simulink model "PubIfDecisionTOS_MDL"  (R2020b)
settings: configuration reference "DspaceConfig" (kept outside this file)
PostLoadFcn:
  | if any(exist('dsrtsu_mdlpostloadfcn', 'file') ~= 0), dsrtsu_mdlpostloadfcn('Execute', bdroot); end
InitFcn:
  | , if any(exist('dsmpb_private', 'file') ~= 0), dsmpb_private('dsmpb_mdlclblib', 'Init', bdroot); end,
undefined symbols (not defined in the file or in its folder): C_TOS_ACCEgoRAxletoFbumplength_m, C_TOS_ACCTargetFront_Flag, C_TOS_AEBJAPedObjDxThre_Val, C_TOS_AEBJAPedObjDyThre_Val, C_TOS_AEBJATargetSize_Val, C_TOS_AEBJAVehObjDxThre_Val, C_TOS_AEBJAVehObjDyThre_Val, C_TOS_AEBJuncPedTargetSize_Val, C_TOS_AEBLatObjDxThre_Val, C_TOS_AEBLatPedDyThre_Val, C_TOS_AEBLatTargetSize_Val, C_TOS_AEBLongTargetInEgoFront_Flag, C_TOS_axAbsGround_Parameter, C_TOS_CameraConfirmedFlag, C_TOS_CNsubjWidth, C_TOS_CurrentLaneCoreMinWidth_Val, C_TOS_CutInProb_Val_Zero, C_TOS_CutOutProb_Val_Zero, C_TOS_D2R_Val, C_TOS_DefaultValueObjectToCenterLine_dy, C_TOS_EgoCarWidth_Val, C_TOS_EgoDxRefPoint_m, C_TOS_EgoRAxletoFbumplength_m, C_TOS_HalfWidthVehicle_Con, C_TOS_HWA_CurrentLaneFlag, C_TOS_HWA_LeftLaneFlag, C_TOS_HWA_MovingDir_Vaild, C_TOS_HWA_MovState_Vaild, C_TOS_HWA_RightLaneFlag, C_TOS_LaneLineCourseErrorFront, C_TOS_LaneLineCourseErrorRear, C_TOS_MotorbikeDefaultWidth_m, C_TOS_NumberOfEffectiveTargets, C_TOS_Obj_Age_Val, C_TOS_Objdx_Constraint_Val, C_TOS_ObjectDefaultWidth_m, C_TOS_ObjInCurrentLane_Val, C_TOS_ObjInCurrentLaneValid, C_TOS_ObjInLeftLaneValid, C_TOS_ObjInRightLaneValid, C_TOS_ObjNotInCurrentLane_Val, C_TOS_ObjNotREElementType, C_TOS_ObjPredictDis_dy_ConstantVal_Zeros, C_TOS_ObjToCenterLine_ConstantVal_Zeros, C_TOS_OFMObjIDInvilad_Val, C_TOS_PIL_LatDisCons_Val_zero, C_TOS_PIL_ObjectCutInFlag_b, C_TOS_PIL_ObjectCutOutFlag_b, C_TOS_PIL_ObjLaneProb_al_Val, C_TOS_PP_ObjFusType_FC_Confirm_b, C_TOS_PP_ObjFusType_FC_FR_Confirm_b, C_TOS_PP_ObjFusType_FR_Confirm_b, C_TOS_RE_80BoolDefault_Val, C_TOS_RE_80Single181Default_Val, C_TOS_RE_80Single255Default_Val, C_TOS_RE_80Uint8Default_Val, C_TOS_RE_D2R, C_TOS_RE_D_180_Val, C_TOS_RE_InvalidObjectID_Val, C_TOS_RE_InvalidTargetChainDir_Val ... (+142)
libraries: simulink x1650, TOS_LIB x361, canfdmsglib x14
(part 25 of 69)

== system PubIfDecisionTOS_MDL/TOS_20201112/TOS_2012080320/PP1128/AAT-AdditionalAttributes/PP_SignalProcessing/PP_SignalProcessing/MovingState_SignalProcessing/MovingState_SignalProcessing_V2011120315 ==
  Object_MovingState : Inport
  Compare To Constant : simulink/Logic and Bit Operations/Compare To Constant  relop===  const=OFM_OBJ_MOVINGSTATE_E.MOVING  OutDataTypeStr=boolean
      settings: AttributesFormatString=OFM_OBJ_MOVINGSTATE_E.MOVING = 2
  Compare To Constant1 : simulink/Logic and Bit Operations/Compare To Constant  relop===  const=OFM_OBJ_MOVINGSTATE_E.MOVING_SLOWLY  OutDataTypeStr=boolean
      settings: AttributesFormatString=OFM_OBJ_MOVINGSTATE_E.MOVING_SLOWLY = 5
  Compare To Constant2 : simulink/Logic and Bit Operations/Compare To Constant  relop===  const=OFM_OBJ_MOVINGSTATE_E.STATIONARY  OutDataTypeStr=boolean
      settings: AttributesFormatString=OFM_OBJ_MOVINGSTATE_E.STATIONARY = 3
  Compare To Constant3 : simulink/Logic and Bit Operations/Compare To Constant  relop===  const=OFM_OBJ_MOVINGSTATE_E.STOPPED  OutDataTypeStr=boolean
      settings: AttributesFormatString=OFM_OBJ_MOVINGSTATE_E.STOPPED = 4
  Data Type Conversion : DataTypeConversion  OutDataTypeStr=Enum: OFM_OBJ_MOVINGSTATE_E
  Data Type Conversion1 : DataTypeConversion  OutDataTypeStr=uint8
  Enumerated Constant : simulink/Sources/Enumerated Constant  OutDataTypeStr=Enum: ObjectMovingState_AEB_E  Value=ObjectMovingState_AEB_E.Moving  SampleTime=inf
      settings: AttributesFormatString=ObjectMovingState.Moving =2
  Enumerated Constant1 : simulink/Sources/Enumerated Constant  OutDataTypeStr=Enum: ObjectMovingState_AEB_E  Value=ObjectMovingState_AEB_E.Still  SampleTime=inf
      settings: AttributesFormatString=ObjectMovingState.Still = 1
  Enumerated Constant2 : simulink/Sources/Enumerated Constant  OutDataTypeStr=Enum: ObjectMovingState_AEB_E  Value=ObjectMovingState_AEB_E.Stopped  SampleTime=inf
      settings: AttributesFormatString=ObjectMovingState.Stopped = 3
  Enumerated Constant3 : simulink/Sources/Enumerated Constant  OutDataTypeStr=Enum: ObjectMovingState_AEB_E  Value=ObjectMovingState_AEB_E.UnknownState  SampleTime=inf
      settings: AttributesFormatString=ObjectMovingState.UnknownState = 0
  Logical Operator : Logic  Operator=OR  AllPortsSameDT=off  OutDataTypeStr=boolean
  Switch : Switch  Criteria=u2 ~= 0
  Switch1 : Switch  Criteria=u2 ~= 0
  Switch2 : Switch  Criteria=u2 ~= 0
  PP_MovingStateSignalProcessing : Outport
  wires:
  Switch1/1 -> Switch/3
  Switch2/1 -> Switch1/3
  Enumerated Constant2/1 -> Switch2/1
  Compare To Constant3/1 -> Switch2/2
  Enumerated Constant1/1 -> Switch1/1
  Compare To Constant2/1 -> Switch1/2
  Enumerated Constant/1 -> Switch/1
  Logical Operator/1 -> Switch/2
  Compare To Constant1/1 -> Logical Operator/2
  Compare To Constant/1 -> Logical Operator/1
  Data Type Conversion/1 -> Compare To Constant3/1, Compare To Constant2/1, Compare To Constant1/1, Compare To Constant/1
  Object_MovingState/1 -> Data Type Conversion/1
  Data Type Conversion1/1 -> PP_MovingStateSignalProcessing/1
  Switch/1 -> Data Type Conversion1/1
  Enumerated Constant3/1 -> Switch2/3

== system PubIfDecisionTOS_MDL/TOS_20201112/TOS_2012080320/PP1128/AAT-AdditionalAttributes/PP_SignalProcessing/PP_SignalProcessing/MovingState_SignalProcessing/MovingState_SignalProcessing_V2011130316 ==
  Object_MovingState : Inport
  Compare To Constant : simulink/Logic and Bit Operations/Compare To Constant  relop===  const=OFM_OBJ_MOVINGSTATE_E.MOVING  OutDataTypeStr=boolean
      settings: AttributesFormatString=OFM_OBJ_MOVINGSTATE_E.MOVING = 2
  Compare To Constant1 : simulink/Logic and Bit Operations/Compare To Constant  relop===  const=OFM_OBJ_MOVINGSTATE_E.MOVING_SLOWLY  OutDataTypeStr=boolean
      settings: AttributesFormatString=OFM_OBJ_MOVINGSTATE_E.MOVING_SLOWLY = 5
  Compare To Constant2 : simulink/Logic and Bit Operations/Compare To Constant  relop===  const=OFM_OBJ_MOVINGSTATE_E.STATIONARY  OutDataTypeStr=boolean
      settings: AttributesFormatString=OFM_OBJ_MOVINGSTATE_E.STATIONARY = 3
  Compare To Constant3 : simulink/Logic and Bit Operations/Compare To Constant  relop===  const=OFM_OBJ_MOVINGSTATE_E.STOPPED  OutDataTypeStr=boolean
      settings: AttributesFormatString=OFM_OBJ_MOVINGSTATE_E.STOPPED = 4
  Compare To Constant4 : simulink/Logic and Bit Operations/Compare To Constant  relop===  const=OFM_OBJ_MOVINGSTATE_E.INVALID  OutDataTypeStr=boolean
      settings: AttributesFormatString=OFM_OBJ_MOVINGSTATE_E.INVALID = 0
  Data Type Conversion : DataTypeConversion  OutDataTypeStr=Enum: OFM_OBJ_MOVINGSTATE_E
  Data Type Conversion1 : DataTypeConversion  OutDataTypeStr=uint8
  Enumerated Constant : simulink/Sources/Enumerated Constant  OutDataTypeStr=Enum: ObjectMovingState_E  Value=ObjectMovingState_E.Moving  SampleTime=inf
      settings: AttributesFormatString=ObjectMovingState.Moving =2
  Enumerated Constant1 : simulink/Sources/Enumerated Constant  OutDataTypeStr=Enum: ObjectMovingState_E  Value=ObjectMovingState_E.Still  SampleTime=inf
      settings: AttributesFormatString=ObjectMovingState.Still = 3
  Enumerated Constant2 : simulink/Sources/Enumerated Constant  OutDataTypeStr=Enum: ObjectMovingState_E  Value=ObjectMovingState_E.Stopped  SampleTime=inf
      settings: AttributesFormatString=ObjectMovingState.Stopped = 4
  Enumerated Constant3 : simulink/Sources/Enumerated Constant  OutDataTypeStr=Enum: ObjectMovingState_E  Value=ObjectMovingState_E.UnknownState  SampleTime=inf
      settings: AttributesFormatString=ObjectMovingState.UnknownState = 1
  Enumerated Constant4 : simulink/Sources/Enumerated Constant  OutDataTypeStr=Enum: ObjectMovingState_E  Value=ObjectMovingState_E.invalid  SampleTime=inf
      settings: AttributesFormatString=ObjectMovingState_E.invalid = 0
  Logical Operator : Logic  Operator=OR  AllPortsSameDT=off  OutDataTypeStr=boolean
  Switch{,1..3} (4 alike) : Switch  Criteria=u2 ~= 0
  PP_MovingStateSignalProcessing : Outport
  wires:
  Compare To Constant/1 -> Logical Operator/1
  Switch1/1 -> Switch/3
  Compare To Constant4/1 -> Switch3/2
  Enumerated Constant1/1 -> Switch1/1
  Compare To Constant1/1 -> Logical Operator/2
  Data Type Conversion/1 -> Compare To Constant/1, Compare To Constant2/1, Compare To Constant3/1, Compare To Constant1/1, Compare To Constant4/1
  Object_MovingState/1 -> Data Type Conversion/1
  Compare To Constant2/1 -> Switch1/2
  Enumerated Constant4/1 -> Switch3/1
  Enumerated Constant/1 -> Switch/1
  Switch/1 -> Switch3/3
  Compare To Constant3/1 -> Switch2/2
  Enumerated Constant2/1 -> Switch2/1
  Switch3/1 -> Data Type Conversion1/1
  Enumerated Constant3/1 -> Switch2/3
  Switch2/1 -> Switch1/3
  Logical Operator/1 -> Switch/2
  Data Type Conversion1/1 -> PP_MovingStateSignalProcessing/1

== system PubIfDecisionTOS_MDL/TOS_20201112/TOS_2012080320/PP1128/AAT-AdditionalAttributes/PP_SignalProcessing/PP_SignalProcessing/ObjFusTypeConfirm/FC_FR_other ==
  Object_FusType : Inport
  Enumerated Constant : simulink/Sources/Enumerated Constant  OutDataTypeStr=Enum: OFM_OBJ_FUSTYPE  Value=OFM_OBJ_FUSTYPE.FC_FR  SampleTime=inf
      settings: AttributesFormatString=OFM_OBJ_FUSTYPE.FC_FR = 3
  Enumerated Constant1 : simulink/Sources/Enumerated Constant  OutDataTypeStr=Enum: OFM_OBJ_FUSTYPE  Value=OFM_OBJ_FUSTYPE.FC_FR_CL  SampleTime=inf
      settings: AttributesFormatString=OFM_OBJ_FUSTYPE.FC_FR_CL=7
  Enumerated Constant10 : simulink/Sources/Enumerated Constant  OutDataTypeStr=Enum: OFM_OBJ_FUSTYPE  Value=OFM_OBJ_FUSTYPE.FC_FR_CR_BR  SampleTime=inf
      settings: AttributesFormatString=OFM_OBJ_FUSTYPE.FC_FR_CR_BR=43
  Enumerated Constant11 : simulink/Sources/Enumerated Constant  OutDataTypeStr=Enum: OFM_OBJ_FUSTYPE  Value=OFM_OBJ_FUSTYPE.FC_FR_CL_CR_BR  SampleTime=inf
      settings: AttributesFormatString=OFM_OBJ_FUSTYPE.FC_FR_CL_CR_BR=47
  Enumerated Constant12 : simulink/Sources/Enumerated Constant  OutDataTypeStr=Enum: OFM_OBJ_FUSTYPE  Value=OFM_OBJ_FUSTYPE.FC_FR_BL_BR  SampleTime=inf
      settings: AttributesFormatString=OFM_OBJ_FUSTYPE.FC_FR_BL_BR=51
  Enumerated Constant13 : simulink/Sources/Enumerated Constant  OutDataTypeStr=Enum: OFM_OBJ_FUSTYPE  Value=OFM_OBJ_FUSTYPE.FC_FR_CR_BL_BR  SampleTime=inf
      settings: AttributesFormatString=OFM_OBJ_FUSTYPE.FC_FR_CR_BL_BR=59
  Enumerated Constant14 : simulink/Sources/Enumerated Constant  OutDataTypeStr=Enum: OFM_OBJ_FUSTYPE  Value=OFM_OBJ_FUSTYPE.FC_FR_CL_BL_BR  SampleTime=inf
      settings: AttributesFormatString=OFM_OBJ_FUSTYPE.FC_FR_CL_BL_BR=55
  Enumerated Constant15 : simulink/Sources/Enumerated Constant  OutDataTypeStr=Enum: OFM_OBJ_FUSTYPE  Value=OFM_OBJ_FUSTYPE.FC_FR_CL_CR_BL_BR  SampleTime=inf
      settings: AttributesFormatString=OFM_OBJ_FUSTYPE.FC_FR_CL_CR_BL_BR=63
  Enumerated Constant2 : simulink/Sources/Enumerated Constant  OutDataTypeStr=Enum: OFM_OBJ_FUSTYPE  Value=OFM_OBJ_FUSTYPE.FC_FR_CR  SampleTime=inf
      settings: AttributesFormatString=OFM_OBJ_FUSTYPE.FC_FR_CR=11
  Enumerated Constant3 : simulink/Sources/Enumerated Constant  OutDataTypeStr=Enum: OFM_OBJ_FUSTYPE  Value=OFM_OBJ_FUSTYPE.FC_FR_CL_CR  SampleTime=inf
      settings: AttributesFormatString=OFM_OBJ_FUSTYPE.FC_FR_CL_CR=15
  Enumerated Constant4 : simulink/Sources/Enumerated Constant  OutDataTypeStr=Enum: OFM_OBJ_FUSTYPE  Value=OFM_OBJ_FUSTYPE.FC_FR_BL  SampleTime=inf
      settings: AttributesFormatString=OFM_OBJ_FUSTYPE.FC_FR_BL=19
  Enumerated Constant5 : simulink/Sources/Enumerated Constant  OutDataTypeStr=Enum: OFM_OBJ_FUSTYPE  Value=OFM_OBJ_FUSTYPE.FC_FR_CL_BL  SampleTime=inf
      settings: AttributesFormatString=OFM_OBJ_FUSTYPE.FC_FR_CL_BL=23
  Enumerated Constant6 : simulink/Sources/Enumerated Constant  OutDataTypeStr=Enum: OFM_OBJ_FUSTYPE  Value=OFM_OBJ_FUSTYPE.FC_FR_CR_BL  SampleTime=inf
      settings: AttributesFormatString=OFM_OBJ_FUSTYPE.FC_FR_CR_BL=27
  Enumerated Constant7 : simulink/Sources/Enumerated Constant  OutDataTypeStr=Enum: OFM_OBJ_FUSTYPE  Value=OFM_OBJ_FUSTYPE.FC_FR_CL_CR_BL  SampleTime=inf
      settings: AttributesFormatString=OFM_OBJ_FUSTYPE.FC_FR_CL_CR_BL=31
  Enumerated Constant8 : simulink/Sources/Enumerated Constant  OutDataTypeStr=Enum: OFM_OBJ_FUSTYPE  Value=OFM_OBJ_FUSTYPE.FC_FR_BR  SampleTime=inf
      settings: AttributesFormatString=OFM_OBJ_FUSTYPE.FC_FR_BR=35
  Enumerated Constant9 : simulink/Sources/Enumerated Constant  OutDataTypeStr=Enum: OFM_OBJ_FUSTYPE  Value=OFM_OBJ_FUSTYPE.FC_FR_CL_BR  SampleTime=inf
      settings: AttributesFormatString=OFM_OBJ_FUSTYPE.FC_FR_CL_BR=39
  Logical Operator15 : Logic  Operator=OR  Inputs=16  AllPortsSameDT=off  OutDataTypeStr=boolean
  Relational Operator{1..16} (16 alike) : RelationalOperator  Operator===  OutDataTypeStr=boolean  RndMeth=Nearest
  FC_FR_other : Outport
  wires:
  Object_FusType/1 -> Relational Operator14/1, Relational Operator12/1, Relational Operator3/1, Relational Operator1/1, Relational Operator2/1, Relational Operator4/1, Relational Operator7/1, Relational Operator5/1, Relational Operator6/1, Relational Operator8/1, Relational Operator11/1, Relational Operator9/1, Relational Operator10/1, Relational Operator16/1, Relational Operator15/1, Relational Operator13/1
  Enumerated Constant1/1 -> Relational Operator12/2
  Enumerated Constant2/1 -> Relational Operator13/2
  Enumerated Constant3/1 -> Relational Operator15/2
  Logical Operator15/1 -> FC_FR_other/1
  Enumerated Constant/1 -> Relational Operator14/2
  Enumerated Constant4/1 -> Relational Operator3/2
  Enumerated Constant7/1 -> Relational Operator4/2
  Enumerated Constant6/1 -> Relational Operator2/2
  Enumerated Constant5/1 -> Relational Operator1/2
  Enumerated Constant9/1 -> Relational Operator5/2
  Enumerated Constant10/1 -> Relational Operator6/2
  Enumerated Constant11/1 -> Relational Operator8/2
  Enumerated Constant8/1 -> Relational Operator7/2
  Enumerated Constant12/1 -> Relational Operator11/2
  Enumerated Constant15/1 -> Relational Operator16/2
  Enumerated Constant13/1 -> Relational Operator10/2
  Enumerated Constant14/1 -> Relational Operator9/2
  Relational Operator14/1 -> Logical Operator15/1
  Relational Operator12/1 -> Logical Operator15/2
  Relational Operator13/1 -> Logical Operator15/3
  Relational Operator15/1 -> Logical Operator15/4
  Relational Operator3/1 -> Logical Operator15/5
  Relational Operator1/1 -> Logical Operator15/6
  Relational Operator2/1 -> Logical Operator15/7
  Relational Operator4/1 -> Logical Operator15/8
  Relational Operator7/1 -> Logical Operator15/9
  Relational Operator5/1 -> Logical Operator15/10
  Relational Operator6/1 -> Logical Operator15/11
  Relational Operator8/1 -> Logical Operator15/12
  Relational Operator11/1 -> Logical Operator15/13
  Relational Operator9/1 -> Logical Operator15/14
  Relational Operator10/1 -> Logical Operator15/15
  Relational Operator16/1 -> Logical Operator15/16

== system PubIfDecisionTOS_MDL/TOS_20201112/TOS_2012080320/PP1128/AAT-AdditionalAttributes/PP_SignalProcessing/PP_SignalProcessing/ObjFusTypeConfirm/FC_other ==
  Object_FusType : Inport
  Enumerated Constant : simulink/Sources/Enumerated Constant  OutDataTypeStr=Enum: OFM_OBJ_FUSTYPE  Value=OFM_OBJ_FUSTYPE.FC_FR  SampleTime=inf
      settings: AttributesFormatString=OFM_OBJ_FUSTYPE.FC_FR = 3
  Enumerated Constant1 : simulink/Sources/Enumerated Constant  OutDataTypeStr=Enum: OFM_OBJ_FUSTYPE  Value=OFM_OBJ_FUSTYPE.FC_FR_CL  SampleTime=inf
      settings: AttributesFormatString=OFM_OBJ_FUSTYPE.FC_FR_CL=7
  Enumerated Constant10 : simulink/Sources/Enumerated Constant  OutDataTypeStr=Enum: OFM_OBJ_FUSTYPE  Value=OFM_OBJ_FUSTYPE.FC_FR_CR_BR  SampleTime=inf
      settings: AttributesFormatString=OFM_OBJ_FUSTYPE.FC_FR_CR_BR=43
  Enumerated Constant11 : simulink/Sources/Enumerated Constant  OutDataTypeStr=Enum: OFM_OBJ_FUSTYPE  Value=OFM_OBJ_FUSTYPE.FC_FR_CL_CR_BR  SampleTime=inf
      settings: AttributesFormatString=OFM_OBJ_FUSTYPE.FC_FR_CL_CR_BR=47
  Enumerated Constant12 : simulink/Sources/Enumerated Constant  OutDataTypeStr=Enum: OFM_OBJ_FUSTYPE  Value=OFM_OBJ_FUSTYPE.FC_FR_BL_BR  SampleTime=inf
      settings: AttributesFormatString=OFM_OBJ_FUSTYPE.FC_FR_BL_BR=51
  Enumerated Constant13 : simulink/Sources/Enumerated Constant  OutDataTypeStr=Enum: OFM_OBJ_FUSTYPE  Value=OFM_OBJ_FUSTYPE.FC_FR_CR_BL_BR  SampleTime=inf
      settings: AttributesFormatString=OFM_OBJ_FUSTYPE.FC_FR_CR_BL_BR=59
  Enumerated Constant14 : simulink/Sources/Enumerated Constant  OutDataTypeStr=Enum: OFM_OBJ_FUSTYPE  Value=OFM_OBJ_FUSTYPE.FC_FR_CL_BL_BR  SampleTime=inf
      settings: AttributesFormatString=OFM_OBJ_FUSTYPE.FC_FR_CL_BL_BR=55
  Enumerated Constant15 : simulink/Sources/Enumerated Constant  OutDataTypeStr=Enum: OFM_OBJ_FUSTYPE  Value=OFM_OBJ_FUSTYPE.FC_FR_CL_CR_BL_BR  SampleTime=inf
      settings: AttributesFormatString=OFM_OBJ_FUSTYPE.FC_FR_CL_CR_BL_BR=63
  Enumerated Constant16 : simulink/Sources/Enumerated Constant  OutDataTypeStr=Enum: OFM_OBJ_FUSTYPE  Value=OFM_OBJ_FUSTYPE.FC_CL  SampleTime=inf
      settings: AttributesFormatString=OFM_OBJ_FUSTYPE.FC_CL = 5
  Enumerated Constant17 : simulink/Sources/Enumerated Constant  OutDataTypeStr=Enum: OFM_OBJ_FUSTYPE  Value=OFM_OBJ_FUSTYPE.FC_CL_CR_BL  SampleTime=inf
      settings: AttributesFormatString=OFM_OBJ_FUSTYPE.FC_CL_CR_BL = 29
  Enumerated Constant18 : simulink/Sources/Enumerated Constant  OutDataTypeStr=Enum: OFM_OBJ_FUSTYPE  Value=OFM_OBJ_FUSTYPE.FC_CL_BR  SampleTime=inf
      settings: AttributesFormatString=OFM_OBJ_FUSTYPE.FC_CL_BR = 37
  Enumerated Constant19 : simulink/Sources/Enumerated Constant  OutDataTypeStr=Enum: OFM_OBJ_FUSTYPE  Value=OFM_OBJ_FUSTYPE.FC_CL_CR_BR  SampleTime=inf
      settings: AttributesFormatString=OFM_OBJ_FUSTYPE.FC_CL_CR_BR = 45
  Enumerated Constant2 : simulink/Sources/Enumerated Constant  OutDataTypeStr=Enum: OFM_OBJ_FUSTYPE  Value=OFM_OBJ_FUSTYPE.FC_FR_CR  SampleTime=inf
      settings: AttributesFormatString=OFM_OBJ_FUSTYPE.FC_FR_CR=11
  Enumerated Constant20 : simulink/Sources/Enumerated Constant  OutDataTypeStr=Enum: OFM_OBJ_FUSTYPE  Value=OFM_OBJ_FUSTYPE.FC_CL_BL_BR  SampleTime=inf
      settings: AttributesFormatString=OFM_OBJ_FUSTYPE.FC_CL_BL_BR = 53
  Enumerated Constant21 : simulink/Sources/Enumerated Constant  OutDataTypeStr=Enum: OFM_OBJ_FUSTYPE  Value=OFM_OBJ_FUSTYPE.FC_CL_CR  SampleTime=inf
      settings: AttributesFormatString=OFM_OBJ_FUSTYPE.FC_CL_CR = 13
  Enumerated Constant22 : simulink/Sources/Enumerated Constant  OutDataTypeStr=Enum: OFM_OBJ_FUSTYPE  Value=OFM_OBJ_FUSTYPE.FC_CL_CR_BL_BR  SampleTime=inf
      settings: AttributesFormatString=OFM_OBJ_FUSTYPE.FC_CL_CR_BL_BR = 61
  Enumerated Constant23 : simulink/Sources/Enumerated Constant  OutDataTypeStr=Enum: OFM_OBJ_FUSTYPE  Value=OFM_OBJ_FUSTYPE.FC_CL_BL  SampleTime=inf
      settings: AttributesFormatString=OFM_OBJ_FUSTYPE.FC_CL_BL = 21
  Enumerated Constant24 : simulink/Sources/Enumerated Constant  OutDataTypeStr=Enum: OFM_OBJ_FUSTYPE  Value=OFM_OBJ_FUSTYPE.FC_CR  SampleTime=inf
      settings: AttributesFormatString=OFM_OBJ_FUSTYPE.FC_CR = 9
  Enumerated Constant25 : simulink/Sources/Enumerated Constant  OutDataTypeStr=Enum: OFM_OBJ_FUSTYPE  Value=OFM_OBJ_FUSTYPE.FC_CR_BL_BR  SampleTime=inf
      settings: AttributesFormatString=OFM_OBJ_FUSTYPE.FC_CR_BL_BR = 57
  Enumerated Constant26 : simulink/Sources/Enumerated Constant  OutDataTypeStr=Enum: OFM_OBJ_FUSTYPE  Value=OFM_OBJ_FUSTYPE.FC_CR_BL  SampleTime=inf
      settings: AttributesFormatString=OFM_OBJ_FUSTYPE.FC_CR_BL = 25
  Enumerated Constant27 : simulink/Sources/Enumerated Constant  OutDataTypeStr=Enum: OFM_OBJ_FUSTYPE  Value=OFM_OBJ_FUSTYPE.FC_CR_BR  SampleTime=inf
      settings: AttributesFormatString=OFM_OBJ_FUSTYPE.FC_CR_BR = 41
  Enumerated Constant28 : simulink/Sources/Enumerated Constant  OutDataTypeStr=Enum: OFM_OBJ_FUSTYPE  Value=OFM_OBJ_FUSTYPE.FC  SampleTime=inf
      settings: AttributesFormatString=OFM_OBJ_FUSTYPE.FC = 1
  Enumerated Constant29 : simulink/Sources/Enumerated Constant  OutDataTypeStr=Enum: OFM_OBJ_FUSTYPE  Value=OFM_OBJ_FUSTYPE.FC_BL  SampleTime=inf
      settings: AttributesFormatString=OFM_OBJ_FUSTYPE.FC_BL = 17
  Enumerated Constant3 : simulink/Sources/Enumerated Constant  OutDataTypeStr=Enum: OFM_OBJ_FUSTYPE  Value=OFM_OBJ_FUSTYPE.FC_FR_CL_CR  SampleTime=inf
      settings: AttributesFormatString=OFM_OBJ_FUSTYPE.FC_FR_CL_CR=15
  Enumerated Constant30 : simulink/Sources/Enumerated Constant  OutDataTypeStr=Enum: OFM_OBJ_FUSTYPE  Value=OFM_OBJ_FUSTYPE.FC_BR  SampleTime=inf
      settings: AttributesFormatString=OFM_OBJ_FUSTYPE.FC_BR = 33
  Enumerated Constant31 : simulink/Sources/Enumerated Constant  OutDataTypeStr=Enum: OFM_OBJ_FUSTYPE  Value=OFM_OBJ_FUSTYPE.FC_BL_BR  SampleTime=inf
      settings: AttributesFormatString=OFM_OBJ_FUSTYPE.FC_BL_BR = 49
  Enumerated Constant4 : simulink/Sources/Enumerated Constant  OutDataTypeStr=Enum: OFM_OBJ_FUSTYPE  Value=OFM_OBJ_FUSTYPE.FC_FR_BL  SampleTime=inf
      settings: AttributesFormatString=OFM_OBJ_FUSTYPE.FC_FR_BL=19
  Enumerated Constant5 : simulink/Sources/Enumerated Constant  OutDataTypeStr=Enum: OFM_OBJ_FUSTYPE  Value=OFM_OBJ_FUSTYPE.FC_FR_CL_BL  SampleTime=inf
      settings: AttributesFormatString=OFM_OBJ_FUSTYPE.FC_FR_CL_BL=23
  Enumerated Constant6 : simulink/Sources/Enumerated Constant  OutDataTypeStr=Enum: OFM_OBJ_FUSTYPE  Value=OFM_OBJ_FUSTYPE.FC_FR_CR_BL  SampleTime=inf
      settings: AttributesFormatString=OFM_OBJ_FUSTYPE.FC_FR_CR_BL=27
  Enumerated Constant7 : simulink/Sources/Enumerated Constant  OutDataTypeStr=Enum: OFM_OBJ_FUSTYPE  Value=OFM_OBJ_FUSTYPE.FC_FR_CL_CR_BL  SampleTime=inf
      settings: AttributesFormatString=OFM_OBJ_FUSTYPE.FC_FR_CL_CR_BL=31
  Enumerated Constant8 : simulink/Sources/Enumerated Constant  OutDataTypeStr=Enum: OFM_OBJ_FUSTYPE  Value=OFM_OBJ_FUSTYPE.FC_FR_BR  SampleTime=inf
      settings: AttributesFormatString=OFM_OBJ_FUSTYPE.FC_FR_BR=35
  Enumerated Constant9 : simulink/Sources/Enumerated Constant  OutDataTypeStr=Enum: OFM_OBJ_FUSTYPE  Value=OFM_OBJ_FUSTYPE.FC_FR_CL_BR  SampleTime=inf
      settings: AttributesFormatString=OFM_OBJ_FUSTYPE.FC_FR_CL_BR=39
  Logical Operator30 : Logic  Operator=OR  Inputs=32  AllPortsSameDT=off  OutDataTypeStr=boolean
  Relational Operator{1..32} (32 alike) : RelationalOperator  Operator===  OutDataTypeStr=boolean  RndMeth=Nearest
  FC_other : Outport
  wires:
  Logical Operator30/1 -> FC_other/1
  Enumerated Constant11/1 -> Relational Operator25/2
  Enumerated Constant22/1 -> Relational Operator31/2
  Enumerated Constant28/1 -> Relational Operator28/2
  Enumerated Constant13/1 -> Relational Operator30/2
  Enumerated Constant20/1 -> Relational Operator26/2
  Enumerated Constant12/1 -> Relational Operator24/2
  Enumerated Constant2/1 -> Relational Operator17/2
  Enumerated Constant19/1 -> Relational Operator23/2
  Enumerated Constant6/1 -> Relational Operator1/2
  Enumerated Constant21/1 -> Relational Operator11/2
  Enumerated Constant3/1 -> Relational Operator16/2
  Enumerated Constant27/1 -> Relational Operator21/2
  Enumerated Constant23/1 -> Relational Operator3/2
  Enumerated Constant7/1 -> Relational Operator7/2
  Enumerated Constant/1 -> Relational Operator14/2
  Enumerated Constant26/1 -> Relational Operator6/2
  Enumerated Constant17/1 -> Relational Operator5/2
  Enumerated Constant18/1 -> Relational Operator10/2
  Enumerated Constant5/1 -> Relational Operator4/2
  Enumerated Constant14/1 -> Relational Operator29/2
  Enumerated Constant8/1 -> Relational Operator9/2
  Enumerated Constant25/1 -> Relational Operator27/2
  Enumerated Constant10/1 -> Relational Operator22/2
  Enumerated Constant24/1 -> Relational Operator15/2
  Enumerated Constant29/1 -> Relational Operator18/2
  Object_FusType/1 -> Relational Operator32/1, Relational Operator31/1, Relational Operator30/1, Relational Operator27/1, Relational Operator29/1, Relational Operator26/1, Relational Operator24/1, Relational Operator8/1, Relational Operator25/1, Relational Operator23/1, Relational Operator22/1, Relational Operator21/1, Relational Operator20/1, Relational Operator10/1, Relational Operator9/1, Relational Operator19/1, Relational Operator7/1, Relational Operator5/1, Relational Operator1/1, Relational Operator6/1, Relational Operator4/1, Relational Operator3/1, Relational Operator2/1, Relational Operator18/1, Relational Operator16/1, Relational Operator11/1, Relational Operator17/1, Relational Operator15/1, Relational Operator13/1, Relational Operator12/1, Relational Operator14/1, Relational Operator28/1
  Enumerated Constant9/1 -> Relational Operator20/2
  Enumerated Constant30/1 -> Relational Operator19/2
  Enumerated Constant16/1 -> Relational Operator12/2
  Enumerated Constant31/1 -> Relational Operator8/2
  Enumerated Constant15/1 -> Relational Operator32/2
  Enumerated Constant1/1 -> Relational Operator13/2
  Enumerated Constant4/1 -> Relational Operator2/2
  Relational Operator28/1 -> Logical Operator30/1
  Relational Operator14/1 -> Logical Operator30/2
  Relational Operator12/1 -> Logical Operator30/3
  Relational Operator13/1 -> Logical Operator30/4
  Relational Operator15/1 -> Logical Operator30/5
  Relational Operator17/1 -> Logical Operator30/6
  Relational Operator11/1 -> Logical Operator30/7
  Relational Operator16/1 -> Logical Operator30/8
  Relational Operator18/1 -> Logical Operator30/9
  Relational Operator2/1 -> Logical Operator30/10
  Relational Operator3/1 -> Logical Operator30/11
  Relational Operator4/1 -> Logical Operator30/12
  Relational Operator6/1 -> Logical Operator30/13
  Relational Operator1/1 -> Logical Operator30/14
  Relational Operator5/1 -> Logical Operator30/15
  Relational Operator7/1 -> Logical Operator30/16
  Relational Operator19/1 -> Logical Operator30/17
  Relational Operator9/1 -> Logical Operator30/18
  Relational Operator10/1 -> Logical Operator30/19
  Relational Operator20/1 -> Logical Operator30/20
  Relational Operator21/1 -> Logical Operator30/21
  Relational Operator22/1 -> Logical Operator30/22
  Relational Operator23/1 -> Logical Operator30/23
  Relational Operator25/1 -> Logical Operator30/24
  Relational Operator8/1 -> Logical Operator30/25
  Relational Operator24/1 -> Logical Operator30/26
  Relational Operator26/1 -> Logical Operator30/27
  Relational Operator29/1 -> Logical Operator30/28
  Relational Operator27/1 -> Logical Operator30/29
  Relational Operator30/1 -> Logical Operator30/30
  Relational Operator31/1 -> Logical Operator30/31
  Relational Operator32/1 -> Logical Operator30/32

== system PubIfDecisionTOS_MDL/TOS_20201112/TOS_2012080320/PP1128/AAT-AdditionalAttributes/PP_SignalProcessing/PP_SignalProcessing/ObjFusTypeConfirm/FR_other ==
  Object_FusType : Inport
  Enumerated Constant63 : simulink/Sources/Enumerated Constant  OutDataTypeStr=Enum: OFM_OBJ_FUSTYPE  Value=OFM_OBJ_FUSTYPE.FR  SampleTime=inf
      settings: AttributesFormatString=OFM_OBJ_FUSTYPE.FR = 2
  Enumerated Constant64 : simulink/Sources/Enumerated Constant  OutDataTypeStr=Enum: OFM_OBJ_FUSTYPE  Value=OFM_OBJ_FUSTYPE.FC_FR  SampleTime=inf
      settings: AttributesFormatString=OFM_OBJ_FUSTYPE.FC_FR = 3
  Enumerated Constant65 : simulink/Sources/Enumerated Constant  OutDataTypeStr=Enum: OFM_OBJ_FUSTYPE  Value=OFM_OBJ_FUSTYPE.FR_CL  SampleTime=inf
      settings: AttributesFormatString=OFM_OBJ_FUSTYPE.FR_CL = 6
  Enumerated Constant66 : simulink/Sources/Enumerated Constant  OutDataTypeStr=Enum: OFM_OBJ_FUSTYPE  Value=OFM_OBJ_FUSTYPE.FC_FR_CL  SampleTime=inf
      settings: AttributesFormatString=OFM_OBJ_FUSTYPE.FC_FR_CL=7
  Enumerated Constant67 : simulink/Sources/Enumerated Constant  OutDataTypeStr=Enum: OFM_OBJ_FUSTYPE  Value=OFM_OBJ_FUSTYPE.FR_CR  SampleTime=inf
      settings: AttributesFormatString=OFM_OBJ_FUSTYPE.FR_CR = 10
  Enumerated Constant68 : simulink/Sources/Enumerated Constant  OutDataTypeStr=Enum: OFM_OBJ_FUSTYPE  Value=OFM_OBJ_FUSTYPE.FC_FR_CR  SampleTime=inf
      settings: AttributesFormatString=OFM_OBJ_FUSTYPE.FC_FR_CR=11
  Enumerated Constant69 : simulink/Sources/Enumerated Constant  OutDataTypeStr=Enum: OFM_OBJ_FUSTYPE  Value=OFM_OBJ_FUSTYPE.FR_CL_CR  SampleTime=inf
      settings: AttributesFormatString=OFM_OBJ_FUSTYPE.FR_CL_CR = 14
  Enumerated Constant70 : simulink/Sources/Enumerated Constant  OutDataTypeStr=Enum: OFM_OBJ_FUSTYPE  Value=OFM_OBJ_FUSTYPE.FC_FR_CL_CR  SampleTime=inf
      settings: AttributesFormatString=OFM_OBJ_FUSTYPE.FC_FR_CL_CR=15
  Enumerated Constant71 : simulink/Sources/Enumerated Constant  OutDataTypeStr=Enum: OFM_OBJ_FUSTYPE  Value=OFM_OBJ_FUSTYPE.FR_BL  SampleTime=inf
      settings: AttributesFormatString=OFM_OBJ_FUSTYPE.FR_BL = 18
  Enumerated Constant72 : simulink/Sources/Enumerated Constant  OutDataTypeStr=Enum: OFM_OBJ_FUSTYPE  Value=OFM_OBJ_FUSTYPE.FC_FR_BL  SampleTime=inf
      settings: AttributesFormatString=OFM_OBJ_FUSTYPE.FC_FR_BL=19
  Enumerated Constant73 : simulink/Sources/Enumerated Constant  OutDataTypeStr=Enum: OFM_OBJ_FUSTYPE  Value=OFM_OBJ_FUSTYPE.FR_CL_BL  SampleTime=inf
      settings: AttributesFormatString=OFM_OBJ_FUSTYPE.FR_CL_BL = 22
  Enumerated Constant74 : simulink/Sources/Enumerated Constant  OutDataTypeStr=Enum: OFM_OBJ_FUSTYPE  Value=OFM_OBJ_FUSTYPE.FC_FR_CL_BL  SampleTime=inf
      settings: AttributesFormatString=OFM_OBJ_FUSTYPE.FC_FR_CL_BL=23
  Enumerated Constant75 : simulink/Sources/Enumerated Constant  OutDataTypeStr=Enum: OFM_OBJ_FUSTYPE  Value=OFM_OBJ_FUSTYPE.FR_CR_BL  SampleTime=inf
      settings: AttributesFormatString=OFM_OBJ_FUSTYPE.FR_CR_BL = 26
  Enumerated Constant76 : simulink/Sources/Enumerated Constant  OutDataTypeStr=Enum: OFM_OBJ_FUSTYPE  Value=OFM_OBJ_FUSTYPE.FC_FR_CR_BL  SampleTime=inf
      settings: AttributesFormatString=OFM_OBJ_FUSTYPE.FC_FR_CR_BL=27
  Enumerated Constant77 : simulink/Sources/Enumerated Constant  OutDataTypeStr=Enum: OFM_OBJ_FUSTYPE  Value=OFM_OBJ_FUSTYPE.FR_CL_CR_BL  SampleTime=inf
      settings: AttributesFormatString=OFM_OBJ_FUSTYPE.FR_CL_CR_BL = 30
  Enumerated Constant78 : simulink/Sources/Enumerated Constant  OutDataTypeStr=Enum: OFM_OBJ_FUSTYPE  Value=OFM_OBJ_FUSTYPE.FC_FR_CL_CR_BL  SampleTime=inf
      settings: AttributesFormatString=OFM_OBJ_FUSTYPE.FC_FR_CL_CR_BL=31
  Enumerated Constant79 : simulink/Sources/Enumerated Constant  OutDataTypeStr=Enum: OFM_OBJ_FUSTYPE  Value=OFM_OBJ_FUSTYPE.FR_BR  SampleTime=inf
      settings: AttributesFormatString=OFM_OBJ_FUSTYPE.FR_BR = 34
  Enumerated Constant80 : simulink/Sources/Enumerated Constant  OutDataTypeStr=Enum: OFM_OBJ_FUSTYPE  Value=OFM_OBJ_FUSTYPE.FC_FR_BR  SampleTime=inf
      settings: AttributesFormatString=OFM_OBJ_FUSTYPE.FC_FR_BR=35
  Enumerated Constant81 : simulink/Sources/Enumerated Constant  OutDataTypeStr=Enum: OFM_OBJ_FUSTYPE  Value=OFM_OBJ_FUSTYPE.FR_CL_BR  SampleTime=inf
      settings: AttributesFormatString=OFM_OBJ_FUSTYPE.FR_CL_BR = 38
  Enumerated Constant82 : simulink/Sources/Enumerated Constant  OutDataTypeStr=Enum: OFM_OBJ_FUSTYPE  Value=OFM_OBJ_FUSTYPE.FC_FR_CL_BR  SampleTime=inf
      settings: AttributesFormatString=OFM_OBJ_FUSTYPE.FC_FR_CL_BR=39
  Enumerated Constant83 : simulink/Sources/Enumerated Constant  OutDataTypeStr=Enum: OFM_OBJ_FUSTYPE  Value=OFM_OBJ_FUSTYPE.FR_CR_BR  SampleTime=inf
      settings: AttributesFormatString=OFM_OBJ_FUSTYPE.FR_CR_BR = 42
  Enumerated Constant84 : simulink/Sources/Enumerated Constant  OutDataTypeStr=Enum: OFM_OBJ_FUSTYPE  Value=OFM_OBJ_FUSTYPE.FC_FR_CR_BR  SampleTime=inf
      settings: AttributesFormatString=OFM_OBJ_FUSTYPE.FC_FR_CR_BR=43
  Enumerated Constant85 : simulink/Sources/Enumerated Constant  OutDataTypeStr=Enum: OFM_OBJ_FUSTYPE  Value=OFM_OBJ_FUSTYPE.FR_CL_CR_BR  SampleTime=inf
      settings: AttributesFormatString=OFM_OBJ_FUSTYPE.FR_CL_CR_BR = 46
  Enumerated Constant86 : simulink/Sources/Enumerated Constant  OutDataTypeStr=Enum: OFM_OBJ_FUSTYPE  Value=OFM_OBJ_FUSTYPE.FC_FR_CL_CR_BR  SampleTime=inf
      settings: AttributesFormatString=OFM_OBJ_FUSTYPE.FC_FR_CL_CR_BR=47
  Enumerated Constant87 : simulink/Sources/Enumerated Constant  OutDataTypeStr=Enum: OFM_OBJ_FUSTYPE  Value=OFM_OBJ_FUSTYPE.FR_BL_BR  SampleTime=inf
      settings: AttributesFormatString=OFM_OBJ_FUSTYPE.FR_BL_BR = 50
  Enumerated Constant88 : simulink/Sources/Enumerated Constant  OutDataTypeStr=Enum: OFM_OBJ_FUSTYPE  Value=OFM_OBJ_FUSTYPE.FC_FR_BL_BR  SampleTime=inf
      settings: AttributesFormatString=OFM_OBJ_FUSTYPE.FC_FR_BL_BR=51
  Enumerated Constant89 : simulink/Sources/Enumerated Constant  OutDataTypeStr=Enum: OFM_OBJ_FUSTYPE  Value=OFM_OBJ_FUSTYPE.FR_CL_BL_BR  SampleTime=inf
      settings: AttributesFormatString=OFM_OBJ_FUSTYPE.FR_CL_BL_BR = 54
  Enumerated Constant90 : simulink/Sources/Enumerated Constant  OutDataTypeStr=Enum: OFM_OBJ_FUSTYPE  Value=OFM_OBJ_FUSTYPE.FC_FR_CL_BL_BR  SampleTime=inf
      settings: AttributesFormatString=OFM_OBJ_FUSTYPE.FC_FR_CL_BL_BR=55
  Enumerated Constant91 : simulink/Sources/Enumerated Constant  OutDataTypeStr=Enum: OFM_OBJ_FUSTYPE  Value=OFM_OBJ_FUSTYPE.FR_CR_BL_BR  SampleTime=inf
      settings: AttributesFormatString=OFM_OBJ_FUSTYPE.FR_CR_BL_BR = 58
  Enumerated Constant92 : simulink/Sources/Enumerated Constant  OutDataTypeStr=Enum: OFM_OBJ_FUSTYPE  Value=OFM_OBJ_FUSTYPE.FC_FR_CR_BL_BR  SampleTime=inf
      settings: AttributesFormatString=OFM_OBJ_FUSTYPE.FC_FR_CR_BL_BR=59
  Enumerated Constant93 : simulink/Sources/Enumerated Constant  OutDataTypeStr=Enum: OFM_OBJ_FUSTYPE  Value=OFM_OBJ_FUSTYPE.FR_CL_CR_BL_BR  SampleTime=inf
      settings: AttributesFormatString=OFM_OBJ_FUSTYPE.FR_CL_CR_BL_BR = 62
  Enumerated Constant94 : simulink/Sources/Enumerated Constant  OutDataTypeStr=Enum: OFM_OBJ_FUSTYPE  Value=OFM_OBJ_FUSTYPE.FC_FR_CL_CR_BL_BR  SampleTime=inf
      settings: AttributesFormatString=OFM_OBJ_FUSTYPE.FC_FR_CL_CR_BL_BR=63
  Logical Operator15 : Logic  Operator=OR  Inputs=32  AllPortsSameDT=off  OutDataTypeStr=boolean
  Relational Operator{16,18..48} (32 alike) : RelationalOperator  Operator===  OutDataTypeStr=boolean  RndMeth=Nearest
  FR_Other : Outport
  wires:
  Logical Operator15/1 -> FR_Other/1
  Enumerated Constant63/1 -> Relational Operator16/2
  Enumerated Constant94/1 -> Relational Operator18/2
  Enumerated Constant64/1 -> Relational Operator19/2
  Enumerated Constant65/1 -> Relational Operator20/2
  Enumerated Constant66/1 -> Relational Operator21/2
  Enumerated Constant70/1 -> Relational Operator25/2
  Enumerated Constant69/1 -> Relational Operator24/2
  Enumerated Constant68/1 -> Relational Operator23/2
  Enumerated Constant67/1 -> Relational Operator22/2
  Enumerated Constant75/1 -> Relational Operator30/2
  Enumerated Constant76/1 -> Relational Operator31/2
  Enumerated Constant77/1 -> Relational Operator32/2
  Enumerated Constant78/1 -> Relational Operator33/2
  Enumerated Constant74/1 -> Relational Operator29/2
  Enumerated Constant73/1 -> Relational Operator28/2
  Enumerated Constant72/1 -> Relational Operator27/2
  Enumerated Constant71/1 -> Relational Operator26/2
  Enumerated Constant87/1 -> Relational Operator42/2
  Enumerated Constant88/1 -> Relational Operator43/2
  Enumerated Constant89/1 -> Relational Operator44/2
  Enumerated Constant90/1 -> Relational Operator45/2
  Enumerated Constant93/1 -> Relational Operator48/2
  Enumerated Constant92/1 -> Relational Operator47/2
  Enumerated Constant91/1 -> Relational Operator46/2
  Object_FusType/1 -> Relational Operator19/1, Relational Operator20/1, Relational Operator21/1, Relational Operator22/1, Relational Operator23/1, Relational Operator24/1, Relational Operator25/1, Relational Operator26/1, Relational Operator27/1, Relational Operator28/1, Relational Operator29/1, Relational Operator30/1, Relational Operator31/1, Relational Operator32/1, Relational Operator33/1, Relational Operator34/1, Relational Operator35/1, Relational Operator36/1, Relational Operator37/1, Relational Operator38/1, Relational Operator39/1, Relational Operator40/1, Relational Operator41/1, Relational Operator42/1, Relational Operator43/1, Relational Operator44/1, Relational Operator45/1, Relational Operator46/1, Relational Operator47/1, Relational Operator48/1, Relational Operator18/1, Relational Operator16/1
  Enumerated Constant83/1 -> Relational Operator38/2
  Enumerated Constant84/1 -> Relational Operator39/2
  Enumerated Constant85/1 -> Relational Operator40/2
  Enumerated Constant86/1 -> Relational Operator41/2
  Enumerated Constant82/1 -> Relational Operator37/2
  Enumerated Constant81/1 -> Relational Operator36/2
  Enumerated Constant80/1 -> Relational Operator35/2
  Enumerated Constant79/1 -> Relational Operator34/2
  Relational Operator16/1 -> Logical Operator15/1
  Relational Operator19/1 -> Logical Operator15/2
  Relational Operator20/1 -> Logical Operator15/3
  Relational Operator21/1 -> Logical Operator15/4
  Relational Operator22/1 -> Logical Operator15/5
  Relational Operator23/1 -> Logical Operator15/6
  Relational Operator24/1 -> Logical Operator15/7
  Relational Operator25/1 -> Logical Operator15/8
  Relational Operator26/1 -> Logical Operator15/9
  Relational Operator27/1 -> Logical Operator15/10
  Relational Operator28/1 -> Logical Operator15/11
  Relational Operator29/1 -> Logical Operator15/12
  Relational Operator30/1 -> Logical Operator15/13
  Relational Operator31/1 -> Logical Operator15/14
  Relational Operator32/1 -> Logical Operator15/15
  Relational Operator33/1 -> Logical Operator15/16
  Relational Operator34/1 -> Logical Operator15/17
  Relational Operator35/1 -> Logical Operator15/18
  Relational Operator36/1 -> Logical Operator15/19
  Relational Operator37/1 -> Logical Operator15/20
  Relational Operator38/1 -> Logical Operator15/21
  Relational Operator39/1 -> Logical Operator15/22
  Relational Operator40/1 -> Logical Operator15/23
  Relational Operator41/1 -> Logical Operator15/24
  Relational Operator42/1 -> Logical Operator15/25
  Relational Operator43/1 -> Logical Operator15/26
  Relational Operator44/1 -> Logical Operator15/27
  Relational Operator45/1 -> Logical Operator15/28
  Relational Operator46/1 -> Logical Operator15/29
  Relational Operator47/1 -> Logical Operator15/30
  Relational Operator48/1 -> Logical Operator15/31
  Relational Operator18/1 -> Logical Operator15/32
